simulink model "Count_Merging_Signals_with_the_Push_Button_Block"  (R2021a)
settings: Solver=VariableStepAuto  StartTime=0.0  StopTime=10.0  RelTol=1e-3
model workspace (MAT data in the model file):
  signal_select = Simulink.Parameter
  signal_select.Value = 1
  signal_select.DataType = 'auto'
  signal_select.Dimensions = [1 1]
libraries: simulink x1
settings Model: Creator=huid  LastModifiedBy=huid

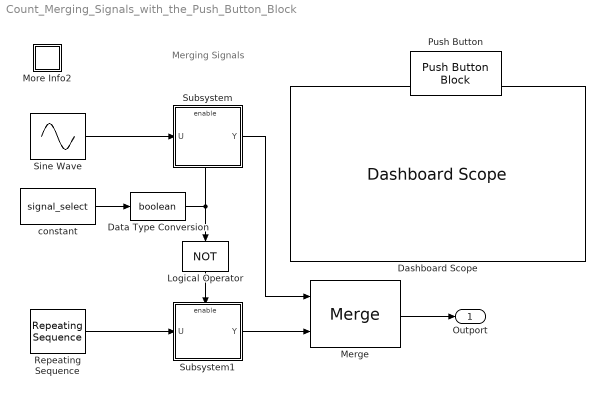
== system Count_Merging_Signals_with_the_Push_Button_Block ==
  note: Merging Signals
  Dashboard Scope : DashboardScope
  Data Type Conversion : DataTypeConversion  OutDataTypeStr=boolean  SaturateOnIntegerOverflow=on  RndMeth=Zero
  Logical Operator : Logic  Operator=NOT  Inputs=1  OutDataTypeStr=boolean
  Merge : Merge
  More Info2 : Subsystem
      settings: OpenFcn=helpview(fullfile(docroot,'simulink','helptargets.map'),'ControlMergingSignalsWithThePushButtonBlockExample')
      mask Display: disp('?')
  Push Button : PushButtonBlock  ButtonText=Signal Select
  Repeating Sequence : simulink/Sources/Repeating Sequence  rep_seq_t=[0 1]  rep_seq_y=[0 2]
  Sine Wave : Sin  Frequency=pi  SampleTime=0
  Subsystem : Subsystem  Tag=MergeExample  TreatAsAtomicUnit=on
  Subsystem1 : Subsystem  Tag=MergeExample  TreatAsAtomicUnit=on
  constant : Constant  Value=signal_select
  Outport : Outport  VectorParamsAs1DForOutWhenUnconnected=off
  wires:
  Sine Wave/1 -> Subsystem/1(U)
  Logical Operator/1 -> Subsystem1/Enable
  Subsystem/1(Y) -> Merge/1
  Data Type Conversion/1 -> Logical Operator/1, Subsystem/Enable
  Merge/1 -> Outport/1
  constant/1 -> Data Type Conversion/1
  Repeating Sequence/1 -> Subsystem1/1(U)
  Subsystem1/1(Y) -> Merge/2

== system Count_Merging_Signals_with_the_Push_Button_Block/More Info2 ==

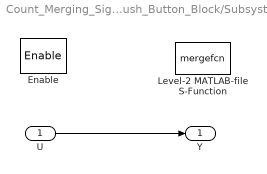
== system Count_Merging_Signals_with_the_Push_Button_Block/Subsystem ==
  U : Inport
  Enable : EnablePort  StatesWhenEnabling=reset
  Level-2 MATLAB-file S-Function : M-S-Function  FunctionName=mergefcn
  Y : Outport  VectorParamsAs1DForOutWhenUnconnected=off
  wires:
  U/1 -> Y/1

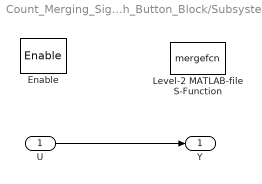
== system Count_Merging_Signals_with_the_Push_Button_Block/Subsystem1 ==
  U : Inport
  Enable : EnablePort  StatesWhenEnabling=reset
  Level-2 MATLAB-file S-Function : M-S-Function  FunctionName=mergefcn
  Y : Outport  VectorParamsAs1DForOutWhenUnconnected=off
  wires:
  U/1 -> Y/1
